simulink model "Recorre_long"  (R2023b)
settings: Solver=VariableStepAuto  StartTime=0.0  StopTime=10.0  RelTol=1e-3
libraries: arduinosensorlib x2
settings Model: Creator=Daniel  LastModifiedBy=Daniel

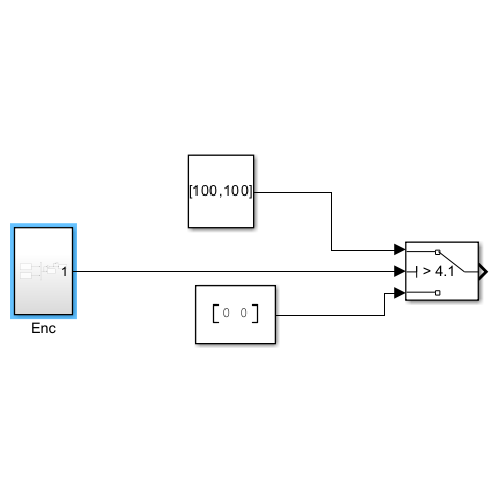
[thumbnail: Simulink's stored preview of the top-level diagram]
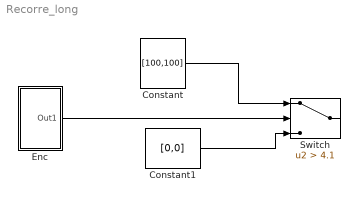
== system Recorre_long ==
  Constant : Constant  Value=[100,100]
  Constant1 : Constant  Value=[0,0]
  Enc : Subsystem
  Switch : Switch  Criteria=u2 > Threshold  Threshold=4.1  SaturateOnIntegerOverflow=off  InputSameDT=off
  wires:
  Constant1/1 -> Switch/3
  Constant/1 -> Switch/1
  Enc/1(Out1) -> Switch/2

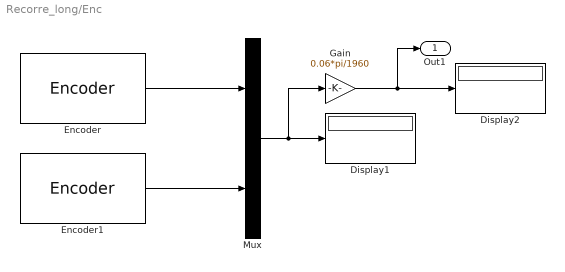
== system Recorre_long/Enc ==
  Display1 : Display
  Display2 : Display
  Encoder : arduinosensorlib/Encoder  InputA=2  InputB=3  Mode=No reset  SampleTime=-1
  Encoder1 : arduinosensorlib/Encoder  InputA=18  InputB=19  Mode=No reset  SampleTime=-1
  Gain : Gain  Gain=0.06*pi/1960
  Mux : Mux  Inputs=2
  Out1 : Outport
  wires:
  Gain/1 -> Out1/1, Display2/1
  Encoder1/1 -> Mux/2
  Mux/1 -> Gain/1, Display1/1
  Encoder/1 -> Mux/1
